simulink model "Part3"  (R2017a)
settings: Solver=VariableStepAuto  StartTime=0.0  StopTime=3  RelTol=1e-3
undefined symbols (not defined in the file): DiscIntNeverNeededParam
libraries: dspstat3 x4, dspsrcs4 x2, dsparch4 x2, commsynccomp2 x2, dspmathops x2
settings Model: Creator=ifaruk  LastModifiedBy=ifaruk

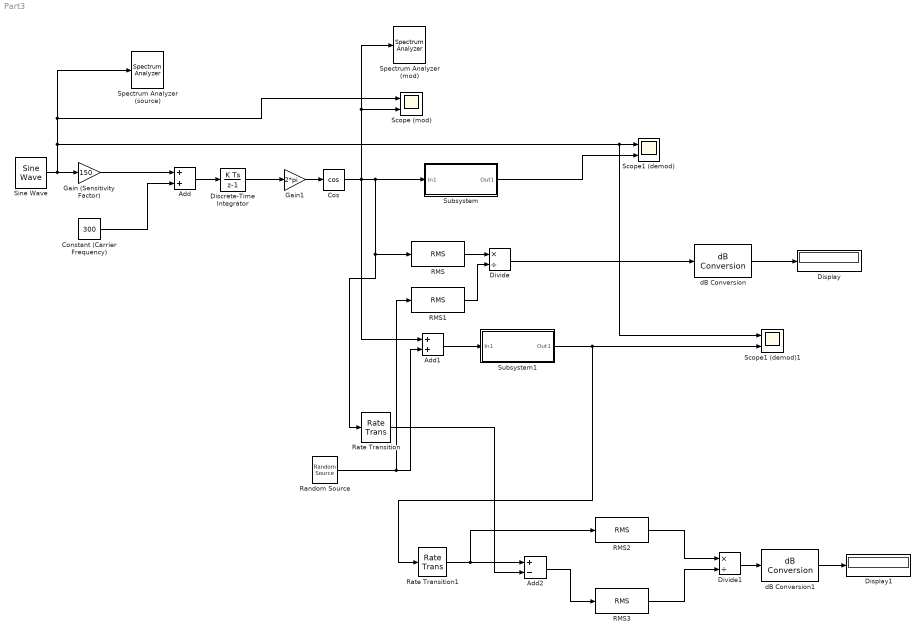
== system Part3 ==
  Add : Sum
  Add1 : Sum
  Add2 : Sum  Inputs=+-
  Constant (Carrier Frequency) : Constant  Value=300
  Cos : Trigonometry  Operator=cos
  Discrete-Time Integrator : DiscreteIntegrator  InitialConditionSetting=State (most efficient)  SampleTime=-1  ICPrevOutput=DiscIntNeverNeededParam  ICPrevScaledInput=DiscIntNeverNeededParam
  Display : Display
  Display1 : Display
  Divide : Product  Inputs=*/
  Divide1 : Product  Inputs=*/
  Gain (Sensitivity Factor) : Gain  Gain=150
  Gain1 : Gain  Gain=2*pi
  RMS{,1..3} (4 alike) : dspstat3/RMS  run=on  directionMode=Each column  dimension=1  InputProcessing=Columns as channels (frame based)  reset_popup=None
  Random Source : dspsrcs4/Random Source  SrcType=Gaussian  NormMethod=Ziggurat  CltLength=12  MinVal=0  MaxVal=1  MeanVal=0  VarVal=0.01  RepMode=Not repeatable  rawSeed=1  IsInherit=off  SampMode=Discrete  SampTime=1e-5  SampFrame=1  DataType=Double  OutComplex=Real  OutputFrames=off
  Rate Transition : RateTransition  OutPortSampleTime=1e-6
  Rate Transition1 : RateTransition  OutPortSampleTime=1e-6
  Scope (mod) : Scope  NumInputPorts=2
  Scope1 (demod) : Scope  NumInputPorts=2
  Scope1 (demod)1 : Scope  NumInputPorts=2
  Sine Wave : dspsrcs4/Sine Wave  Amplitude=1  Frequency=1e-2  Phase=0  SampleMode=Discrete  OutComplex=Real  CompMethod=Trigonometric fcn  TableSize=Speed  SampleTime=1/1e5  SamplesPerFrame=1  ResetState=Restart at time zero  OutputFrames=off  dataType=double  wordLen=16  udDataType=sfix(16)  fracBitsMode=Best precision  numFracBits=15  OutDataTypeStr=double  LastOutDataTypeStr=double
  Spectrum Analyzer (mod) : SpectrumAnalyzer
  Spectrum Analyzer (source) : SpectrumAnalyzer
  Subsystem : Subsystem
  Subsystem1 : Subsystem
  dB Conversion : dspmathops/dB Conversion  dBtype=dB  intype=Amplitude  R=1  fuzz=off
      settings: SourceProductName=DSP System Toolbox
  dB Conversion1 : dspmathops/dB Conversion  dBtype=dB  intype=Amplitude  R=1  fuzz=off
      settings: SourceProductName=DSP System Toolbox
  wires:
  Discrete-Time Integrator/1 -> Gain1/1
  Sine Wave/1 -> Scope (mod)/1, Spectrum Analyzer (source)/1, Scope1 (demod)1/1, Scope1 (demod)/1, Gain (Sensitivity Factor)/1
  Gain (Sensitivity Factor)/1 -> Add/1
  Gain1/1 -> Cos/1
  Constant (Carrier Frequency)/1 -> Add/2
  Add/1 -> Discrete-Time Integrator/1
  Cos/1 -> Add1/1, Rate Transition/1, RMS/1, Subsystem/1(In1), Spectrum Analyzer (mod)/1, Scope (mod)/2
  Subsystem/1(Out1) -> Scope1 (demod)/2
  RMS/1 -> Divide/1
  Divide/1 -> dB Conversion/1
  dB Conversion/1 -> Display/1
  Random Source/1 -> RMS1/1, Add1/2
  RMS1/1 -> Divide/2
  Subsystem1/1(Out1) -> Rate Transition1/1, Scope1 (demod)1/2
  Rate Transition/1 -> Add2/2
  Rate Transition1/1 -> RMS2/1, Add2/1
  Add2/1 -> RMS3/1
  RMS2/1 -> Divide1/1
  RMS3/1 -> Divide1/2
  dB Conversion1/1 -> Display1/1
  Divide1/1 -> dB Conversion1/1
  Add1/1 -> Subsystem1/1(In1)

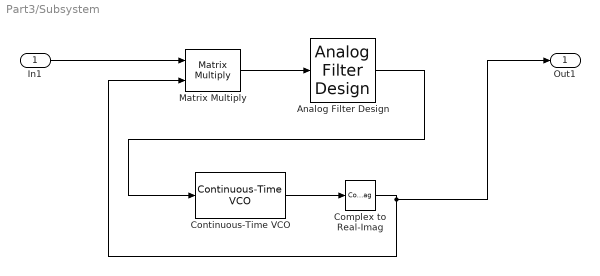
== system Part3/Subsystem ==
  In1 : Inport
  Analog Filter Design : dsparch4/Analog Filter Design  method=Butterworth  filttype=Bandpass  N=8  Wlo=2*pi*8000  Whi=2*pi*10000  Rp=2  Rs=40
  Complex to Real-Imag : ComplexToRealImag  Output=Real
  Continuous-Time VCO : commsynccomp2/Continuous-Time VCO  Ac=1  Fc=100  Kc=50  Ph=0
      settings: SourceProductName=Communications System Toolbox  SourceProductBaseCode=CM
  Matrix Multiply : Product  Multiplication=Matrix(*)
  Out1 : Outport
  wires:
  In1/1 -> Matrix Multiply/1
  Continuous-Time VCO/1 -> Complex to Real-Imag/1
  Complex to Real-Imag/1 -> Out1/1, Matrix Multiply/2
  Matrix Multiply/1 -> Analog Filter Design/1
  Analog Filter Design/1 -> Continuous-Time VCO/1

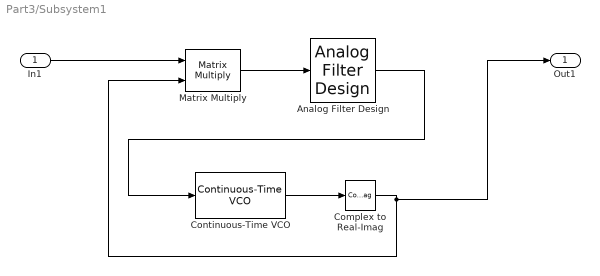
== system Part3/Subsystem1 ==
  In1 : Inport
  Analog Filter Design : dsparch4/Analog Filter Design  method=Butterworth  filttype=Bandpass  N=8  Wlo=2*pi*8000  Whi=2*pi*10000  Rp=2  Rs=40
  Complex to Real-Imag : ComplexToRealImag  Output=Real
  Continuous-Time VCO : commsynccomp2/Continuous-Time VCO  Ac=1  Fc=100  Kc=50  Ph=0
      settings: SourceProductName=Communications System Toolbox  SourceProductBaseCode=CM
  Matrix Multiply : Product  Multiplication=Matrix(*)
  Out1 : Outport
  wires:
  Matrix Multiply/1 -> Analog Filter Design/1
  Analog Filter Design/1 -> Continuous-Time VCO/1
  Complex to Real-Imag/1 -> Out1/1, Matrix Multiply/2
  Continuous-Time VCO/1 -> Complex to Real-Imag/1
  In1/1 -> Matrix Multiply/1
